simulink model "CSTR_T_breach"  (R2021a)
settings: Solver=FixedStepAuto  StartTime=0.0  StopTime=T  FixedStep=Ts  RelTol=1e-3
undefined symbols (not defined in the file): Ts, u0, x0
libraries: simulink x1, sharedTrackingLibrary x1, mpclib x1
settings Model: Creator=The MathWorks, Inc.  LastModifiedBy=ldy
settings SolverCC: AlgebraicLoopSolver=TrustRegion
settings DataIOCC: ReturnWorkspaceOutputs=off
settings DebuggingCC: SFMachineParentedDataDiag=warning  ArithmeticOperatorsInVariantConditions=warning
settings SFSimCC: SimUseLocalCustomCode=off  CustomCodeUndefinedFunction=UseInterfaceOnly
settings RTWCC: RTWUseLocalCustomCode=off

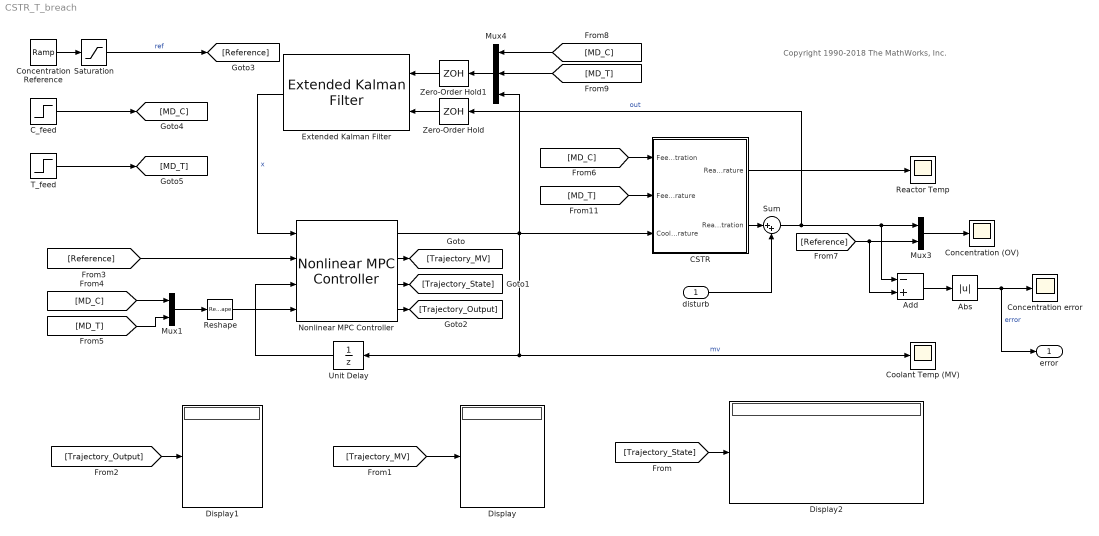
== system CSTR_T_breach ==
  note: Copyright 1990-2018 The MathWorks, Inc.
  disturb : Inport
  Abs : Abs
  Add : Sum  Inputs=-+
  CSTR : Subsystem
  C_feed : Step  Time=10  Before=10  After=10.3  SampleTime=0
  Concentration Reference : simulink/Sources/Ramp  slope=-0.45  start=1  InitialOutput=x0(2)
  Concentration (OV) : Scope
  Concentration error : Scope
  Coolant Temp (MV) : Scope
  Display : Display
  Display1 : Display
  Display2 : Display
  Extended Kalman Filter : sharedTrackingLibrary/Extended Kalman Filter  StateTransitionFcn=exocstrStateFcnDT  HasStateTransitionJacobianFcn=off  HasAdditiveProcessNoise=Additive  ProcessNoise=1e-3  HasTimeVaryingProcessNoise=off  HasStateTransitionFcnExtraArgument=1  InitialState=x0  InitialStateCovariance=1e-3  MeasurementFcn1=exocstrMeasFcn  HasMeasurementJacobianFcn1=off  HasMeasurementEnablePort1=off  HasAdditiveMeasurementNoise1=Additive  MeasurementNoise1=1e-3  HasTimeVaryingMeasurementNoise1=off  HasMeasurementFcnExtraArgument1=0  MeasurementFcn2=myMeasurementFcn  HasMeasurementJacobianFcn2=off  HasMeasurementEnablePort2=off  HasAdditiveMeasurementNoise2=Additive  MeasurementNoise2=1  HasTimeVaryingMeasurementNoise2=off  HasMeasurementFcnExtraArgument2=0  MeasurementFcn3=myMeasurementFcn  HasMeasurementJacobianFcn3=off  HasMeasurementEnablePort3=off  HasAdditiveMeasurementNoise3=Additive  MeasurementNoise3=1  HasTimeVaryingMeasurementNoise3=off  HasMeasurementFcnExtraArgument3=0  MeasurementFcn4=myMeasurementFcn  HasMeasurementJacobianFcn4=off  HasMeasurementEnablePort4=off  HasAdditiveMeasurementNoise4=Additive  MeasurementNoise4=1  HasTimeVaryingMeasurementNoise4=off  HasMeasurementFcnExtraArgument4=0  MeasurementFcn5=myMeasurementFcn  HasMeasurementJacobianFcn5=off  HasMeasurementEnablePort5=off  HasAdditiveMeasurementNoise5=Additive  MeasurementNoise5=1  HasTimeVaryingMeasurementNoise5=off  HasMeasurementFcnExtraArgument5=0  EnableMultirate=off  StateTransitionFcnSampleTime=1  MeasurementFcn1SampleTime=1  MeasurementFcn2SampleTime=1  MeasurementFcn3SampleTime=1  MeasurementFcn4SampleTime=1  MeasurementFcn5SampleTime=1  UseCurrentEstimator=on  OutputStateCovariance=off  DataType=double  SampleTime=Ts  NumberOfMeasurements=1
      settings: SourceProductBaseCode=CT,DR,TF,ID,LP,NV,AR,RO,RR,UV,VE
  Mux1 : Mux  Inputs=2
  Mux3 : Mux  Inputs=2
  Mux4 : Mux  Inputs=3
  Nonlinear MPC Controller : mpclib/Nonlinear MPC Controller  SCDEnableBlockLinearizationSpecification=on  nlmpcobj=nlobj  UseObjectTs=on  UseMEX=off  md_enabled=on  mvtarget_enabled=off  param_enabled=off  cost_enabled=off  mvseq_enabled=on  stateseq_enabled=on  ovseq_enabled=on  slack_enabled=off  status_enabled=off  ov_min=off  ov_max=off  mv_min=off  mv_max=off  mvrate_min=off  mvrate_max=off  state_min=off  state_max=off  ov_weight=off  mv_weight=off  mvrate_weight=off  ecr_weight=off  nlp_initialize=off
  Reactor Temp : Scope
  Reshape : Reshape  OutputDimensionality=Row vector (2-D)
  Saturation : Saturate  UpperLimit=10  LowerLimit=2
  Sum : Sum  Inputs=|++
  T_feed : Step  Time=20  Before=298.15  After=298.15  SampleTime=301
  Unit Delay : UnitDelay  InitialCondition=u0(3)  SampleTime=-1  HasFrameUpgradeWarning=on
  Zero-Order Hold : ZeroOrderHold  SampleTime=Ts
  Zero-Order Hold1 : ZeroOrderHold  SampleTime=Ts
  error : Outport
  wires:
  Nonlinear MPC Controller/1 -> CSTR/3(Coolant Temperature), Coolant Temp (MV)/1, Unit Delay/1, Mux4/3  "mv"
  CSTR/1(Reactor Temperature) -> Reactor Temp/1
  Unit Delay/1 -> Nonlinear MPC Controller/3
  Mux1/1 -> Reshape/1
  Concentration Reference/1 -> Saturation/1
  Mux3/1 -> Concentration (OV)/1
  Extended Kalman Filter/1 -> Nonlinear MPC Controller/1  "x"
  Zero-Order Hold/1 -> Extended Kalman Filter/2
  Mux4/1 -> Zero-Order Hold1/1
  Zero-Order Hold1/1 -> Extended Kalman Filter/1
  Reshape/1 -> Nonlinear MPC Controller/4
  Sum/1 -> Add/1, Mux3/1, Zero-Order Hold/1  "out"
  disturb/1 -> Sum/2
  CSTR/2(Reactor Concentration) -> Sum/1
  Nonlinear MPC Controller/2 -> [Trajectory_MV]
  Nonlinear MPC Controller/3 -> [Trajectory_State]
  [Trajectory_State] -> Display2/1
  [Trajectory_MV] -> Display/1
  Nonlinear MPC Controller/4 -> [Trajectory_Output]
  [Trajectory_Output] -> Display1/1
  Saturation/1 -> [Reference]  "ref"
  [Reference] -> Nonlinear MPC Controller/2
  C_feed/1 -> [MD_C]
  T_feed/1 -> [MD_T]
  [MD_C] -> Mux1/1
  [MD_T] -> Mux1/2
  [MD_C] -> CSTR/1(Feed Concentration)
  [Reference] -> Add/2, Mux3/2
  [MD_C] -> Mux4/1
  [MD_T] -> Mux4/2
  [MD_T] -> CSTR/2(Feed Temperature)
  Add/1 -> Abs/1
  Abs/1 -> error/1, Concentration error/1  "error"

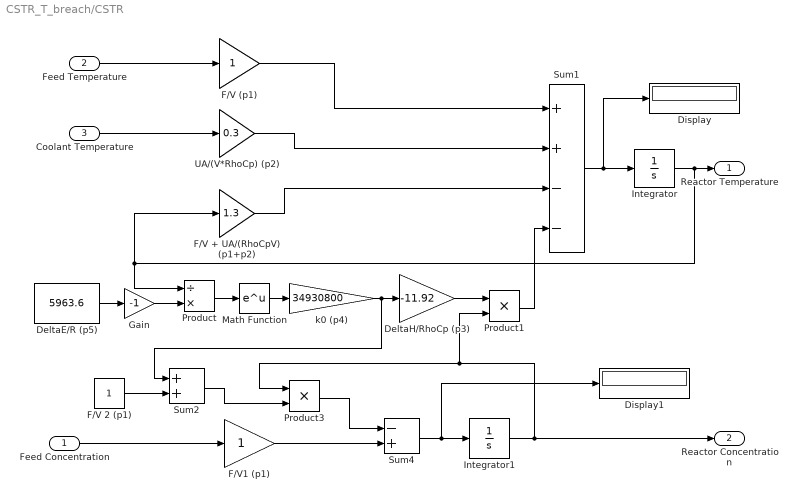
== system CSTR_T_breach/CSTR ==
  Feed Concentration : Inport
  Feed Temperature : Inport  Port=2
  Coolant Temperature : Inport  Port=3
  DeltaE/R (p5) : Constant  Value=5963.6
  DeltaH/RhoCp (p3) : Gain  Gain=-11.92  SaturateOnIntegerOverflow=on  OutDataTypeStr=Inherit: Same as input  ParamDataTypeStr=Inherit: Same as input
  Display : Display
  Display1 : Display
  F/V (p1) : Gain  SaturateOnIntegerOverflow=on  OutDataTypeStr=Inherit: Same as input  ParamDataTypeStr=Inherit: Same as input
  F/V + UA/(RhoCpV) (p1+p2) : Gain  Gain=1.3  SaturateOnIntegerOverflow=on  OutDataTypeStr=Inherit: Same as input  ParamDataTypeStr=Inherit: Same as input
  F/V 2 (p1) : Constant
  F/V1 (p1) : Gain  SaturateOnIntegerOverflow=on  OutDataTypeStr=Inherit: Same as input  ParamDataTypeStr=Inherit: Same as input
  Gain : Gain  Gain=-1
  Integrator : Integrator  InitialCondition=x0(1)  LimitOutput=on  LowerSaturationLimit=0
  Integrator1 : Integrator  InitialCondition=x0(2)  LimitOutput=on  LowerSaturationLimit=0
  Math Function : Math  SignedPower=on  SaturateOnIntegerOverflow=on
  Product : Product  Inputs=/*  InputSameDT=on  RndMeth=Zero  SaturateOnIntegerOverflow=on  OutDataTypeStr=Inherit: Same as first input
  Product1 : Product  InputSameDT=on  RndMeth=Zero  SaturateOnIntegerOverflow=on  OutDataTypeStr=Inherit: Same as first input
  Product3 : Product  InputSameDT=on  RndMeth=Zero  SaturateOnIntegerOverflow=on  OutDataTypeStr=Inherit: Same as first input
  Sum1 : Sum  Inputs=++--  InputSameDT=on  SaturateOnIntegerOverflow=on  OutDataTypeStr=Inherit: Same as first input
  Sum2 : Sum  InputSameDT=on  SaturateOnIntegerOverflow=on  OutDataTypeStr=Inherit: Same as first input
  Sum4 : Sum  Inputs=-+  InputSameDT=on  SaturateOnIntegerOverflow=on  OutDataTypeStr=Inherit: Same as first input
  UA/(V*RhoCp) (p2) : Gain  Gain=0.3  SaturateOnIntegerOverflow=on  OutDataTypeStr=Inherit: Same as input  ParamDataTypeStr=Inherit: Same as input
  k0 (p4) : Gain  Gain=34930800  SaturateOnIntegerOverflow=on  OutDataTypeStr=Inherit: Same as input  ParamDataTypeStr=Inherit: Same as input
  Reactor Temperature : Outport  VectorParamsAs1DForOutWhenUnconnected=off
  Reactor Concentration : Outport  Port=2  VectorParamsAs1DForOutWhenUnconnected=off
  wires:
  F/V (p1)/1 -> Sum1/1
  Sum1/1 -> Display/1, Integrator/1
  Integrator/1 -> Product/1, F/V + UA/(RhoCpV) (p1+p2)/1, Reactor Temperature/1
  UA/(V*RhoCp) (p2)/1 -> Sum1/2
  F/V + UA/(RhoCpV) (p1+p2)/1 -> Sum1/3
  Product/1 -> Math Function/1
  Math Function/1 -> k0 (p4)/1
  DeltaH/RhoCp (p3)/1 -> Product1/1
  Product1/1 -> Sum1/4
  k0 (p4)/1 -> DeltaH/RhoCp (p3)/1, Sum2/1
  DeltaE/R (p5)/1 -> Gain/1
  Product3/1 -> Sum4/1
  Sum4/1 -> Display1/1, Integrator1/1
  Integrator1/1 -> Product1/2, Product3/1, Reactor Concentration/1
  F/V 2 (p1)/1 -> Sum2/2
  F/V1 (p1)/1 -> Sum4/2
  Feed Temperature/1 -> F/V (p1)/1
  Feed Concentration/1 -> F/V1 (p1)/1
  Coolant Temperature/1 -> UA/(V*RhoCp) (p2)/1
  Sum2/1 -> Product3/2
  Gain/1 -> Product/2
